simulink model "Rasmusson"  (R2021b)
settings: Solver=ode15s  StartTime=0.0  StopTime=200  FixedStep=1e-4  MaxStep=0.1  RelTol=1e-6  EnableMultiTasking=on
values from neighbouring files (symbols this model uses):
  Acap = 1.534e-4    (= 0.0001534)    [solver.m]
  aKss = 0.417069e-3    (= 0.000417069)    [solver.m]
  ato_f = 0.265563e-2    (= 0.00265563)    [solver.m]
  ato_s = 0.417069e-3    (= 0.000417069)    [solver.m]
  aur = 0.417069e-3    (= 0.000417069)    [solver.m]
  C2 = 0.124216e-3    (= 0.000124216)    [solver.m]
  C3 = 0.578679e-8    (= 5.78679e-09)    [solver.m]
  C4 = 0.119816e-12    (= 1.19816e-13)    [solver.m]
  Cai = 0.115001    [solver.m]
  CaJSR = 1299.50    (= 1299.5)    [solver.m]
  CaNSR = 1299.50    (= 1299.5)    [solver.m]
  Cao = 1800    [solver.m]
  Cass = 0.115001    [solver.m]
  CK1 = 0.992513e-3    (= 0.000992513)    [solver.m]
  CK2 = 0.641229e-3    (= 0.000641229)    [solver.m]
  Cm = 1.0    (= 1)    [solver.m]
  CMDN_tot = 50.0    (= 50)    [solver.m]
  CNa1 = 0.279132e-3    (= 0.000279132)    [solver.m]
  CNa2 = 0.020752    [solver.m]
  CSQN_tot = 15000.0    (= 15000)    [solver.m]
  ECa_L = 63.0    (= 63)    [solver.m]
  ECl = -40.0    (= -40)    [solver.m]
  F = 96.5    [solver.m]
  GCab = 0.000367    [solver.m]
  GCaL = 0.1729    [solver.m]
  GCl_Ca = 10.0    (= 10)    [solver.m]
  GKr = 0.078    [solver.m]
  GKs = 0.00575    [solver.m]
  GKss = 0.050    (= 0.05)    [solver.m]
  GKtof = pktof(6)    [solver.m]
  GKtos = 0.0    (= 0)    [solver.m]
  GKur = pkslow(6)    [solver.m]
  GNa = 13.0    (= 13)    [solver.m]
  GNab = 0.0026    [solver.m]
  HTRPN_tot = 140.0    (= 140)    [solver.m]
  HTRPNCa = 125.290    (= 125.29)    [solver.m]
  I1 = 0.497923e-18    (= 4.97923e-19)    [solver.m]
  I1Na = 0.673345e-6    (= 6.73345e-07)    [solver.m]
  I2 = 0.345847e-13    (= 3.45847e-14)    [solver.m]
  I2Na = 0.155787e-8    (= 1.55787e-09)    [solver.m]
  I3 = 0.185106e-13    (= 1.85106e-14)    [solver.m]
  ICaL_max = 7.0    (= 7)    [solver.m]
  ICNa2 = 0.0113879    [solver.m]
  ICNa3 = 0.342780    (= 0.34278)    [solver.m]
  IFNa = 0.153176e-3    (= 0.000153176)    [solver.m]
  IK = 0.319129e-4    (= 3.19129e-05)    [solver.m]
  iKss = 1.0    (= 1)    [solver.m]
  INaK_max = 0.88    [solver.m]
  Ip_Ca_max = 1.0    (= 1)    [solver.m]
  ito_f = 0.999977    [solver.m]
  ito_s = 0.998543    [solver.m]
  iur = 0.998543    [solver.m]
  ka1 = 0.006075    [solver.m]
  ka2 = 0.07125    [solver.m]
  kb = 0.036778    [solver.m]
  kb1 = 0.00405    [solver.m]
  kb2 = 0.965    [solver.m]
  kc1 = 0.009    [solver.m]
  kc2 = 0.0008    [solver.m]
  kf = 0.023761    [solver.m]
  khtrpn1 = 0.00237    [solver.m]
  khtrpn2 = 3.2e-5    (= 3.2e-05)    [solver.m]
  Ki = 143720    [solver.m]
  kltrpn1 = 0.0327    [solver.m]
  kltrpn2 = 0.0196    [solver.m]
  Km_Ca = 1380    [solver.m]
  Km_Cl = 10.0    (= 10)    [solver.m]
  Km_CMDN = 0.238    [solver.m]
  Km_CSQN = 800.0    (= 800)    [solver.m]
  Km_Ko = 1500    [solver.m]
  Km_Na = 87500    [solver.m]
  Km_Nai = 21000    [solver.m]
  Km_p_Ca = 0.5    [solver.m]
  Km_up = 0.5    [solver.m]
  kNaCa = 292.8    [solver.m]
  Ko = 5400    [solver.m]
  Kpc_half = 20.0    (= 20)    [solver.m]
  Kpc_max = 0.23324    [solver.m]
  Kpcb = 0.0005    [solver.m]
  ksat = 0.1    [solver.m]
  LTRPN_tot = 70.0    (= 70)    [solver.m]
  LTRPNCa = 11.2684    [solver.m]
  Nai = 14237.1    [solver.m]
  Nao = 140000    [solver.m]
  nKs = 0.262753e-3    (= 0.000262753)    [solver.m]
  nu1 = 4.5    [solver.m]
  nu2 = 1.74e-5    (= 1.74e-05)    [solver.m]
  nu3 = 0.45    [solver.m]
  O = 0.930308e-18    (= 9.30308e-19)    [solver.m]
  OK = 0.175298e-3    (= 0.000175298)    [solver.m]
  ONa = 0.713483e-6    (= 7.13483e-07)    [solver.m]
  PC2 = 0.167740e-3    (= 0.00016774)    [solver.m]
  pkslow = kslow_param_wt(best_KslowWt_idx, :)    [solver.m]
  pktof = to_param_ko(best_toKo_idx, :)    [solver.m]
  PO1 = 0.149102e-4    (= 1.49102e-05)    [solver.m]
  PO2 = 0.951726e-10    (= 9.51726e-11)    [solver.m]
  PRyR = 0.0    (= 0)    [solver.m]
  R = 8.314    [solver.m]
  T = 298    [solver.m]
  tautr = 20.0    (= 20)    [solver.m]
  tauxfer = 8.0    (= 8)    [solver.m]
  V = -50:10:50    [result_analysis.m]    (also in solver.m = -82.4202)
  VJSR = 0.12e-6    (= 1.2e-07)    [solver.m]
  Vmyo = 25.84e-6    (= 2.584e-05)    [solver.m]
  VNSR = 2.098e-6    (= 2.098e-06)    [solver.m]
  Vss = 1.485e-9    (= 1.485e-09)    [solver.m]
  yita = 0.35    [solver.m]
(part 2 of 2)

== system Rasmusson/Concentrations/Caconcentration/Ryanodine_receptors/PO2 ==
  note: A20
  Fcn : Fcn  Expr=u*u*u
  Integrator : Integrator  InitialConditionSource=external  InitialCondition=0.951726e-10
  PO2 : Constant  Value=PO2
  Product : Product  Inputs=3  RndMeth=Zero
  Product1 : Product  RndMeth=Zero
  Subtract : Sum  Inputs=+-
  kb+ : Constant  Value=kb1
  kb- : Constant  Value=kb2
  tag scope: PO2=global
  wires:
  Subtract/1 -> Integrator/1
  Integrator/1 -> [PO2], Product1/2
  Product/1 -> Subtract/1
  Product1/1 -> Subtract/2
  Fcn/1 -> Product/2
  kb+/1 -> Product/1
  [Cass] -> Fcn/1
  [PO1] -> Product/3
  kb-/1 -> Product1/1
  PO2/1 -> Integrator/2

== system Rasmusson/Ionic currents/ICaL/O/C1 ==
  note: A24
  Add : Sum  Inputs=+-------
  Constant : Constant
  tag scope: C1=global
  wires:
  Add/1 -> [C1]
  Constant/1 -> Add/1
  [O] -> Add/2
  [C2] -> Add/3
  [C3] -> Add/4
  [C4] -> Add/5
  [I1] -> Add/6
  [I2] -> Add/7
  [I3] -> Add/8

== system Rasmusson/Ionic currents/ICaL/O/C2 ==
  note: A25
  Add : Sum  Inputs=++--
  C2 : Constant  Value=C2
  Gain : Gain  Gain=4
  Gain1 : Gain  Gain=2
  Gain2 : Gain  Gain=3
  Integrator : Integrator  InitialConditionSource=external  InitialCondition=0.124216e-3
  Product{,1..3} (4 alike) : Product  RndMeth=Zero
  tag scope: C2=global
  wires:
  Add/1 -> Integrator/1
  Gain/1 -> Add/1
  Product/1 -> Gain/1
  [alpha] -> Product/1, Product3/1
  [C1] -> Product/2
  [beta] -> Product1/1, Product2/1
  [C3] -> Product1/2
  Product1/1 -> Gain1/1
  Gain1/1 -> Add/2
  Product2/1 -> Add/3
  Integrator/1 -> [C2], Product2/2, Product3/2
  Product3/1 -> Gain2/1
  Gain2/1 -> Add/4
  C2/1 -> Integrator/2

== system Rasmusson/Ionic currents/ICaL/O/C3 ==
  note: A26
  Add : Sum  Inputs=++--
  C3 : Constant  Value=C3
  Gain : Gain  Gain=3
  Gain1 : Gain  Gain=3
  Gain2 : Gain  Gain=2
  Gain3 : Gain  Gain=2
  Integrator : Integrator  InitialConditionSource=external  InitialCondition=0.578679e-8
  Product{,1..3} (4 alike) : Product  RndMeth=Zero
  tag scope: C3=global
  wires:
  Add/1 -> Integrator/1
  Gain/1 -> Add/1
  Product/1 -> Gain/1
  [alpha] -> Product/1, Product3/1
  [C2] -> Product/2
  [beta] -> Product1/1, Product2/1
  [C4] -> Product1/2
  Product1/1 -> Gain1/1
  Gain1/1 -> Add/2
  Product2/1 -> Gain2/1
  Gain2/1 -> Add/3
  Product3/1 -> Gain3/1
  Gain3/1 -> Add/4
  C3/1 -> Integrator/2
  Integrator/1 -> [C3], Product3/2, Product2/2

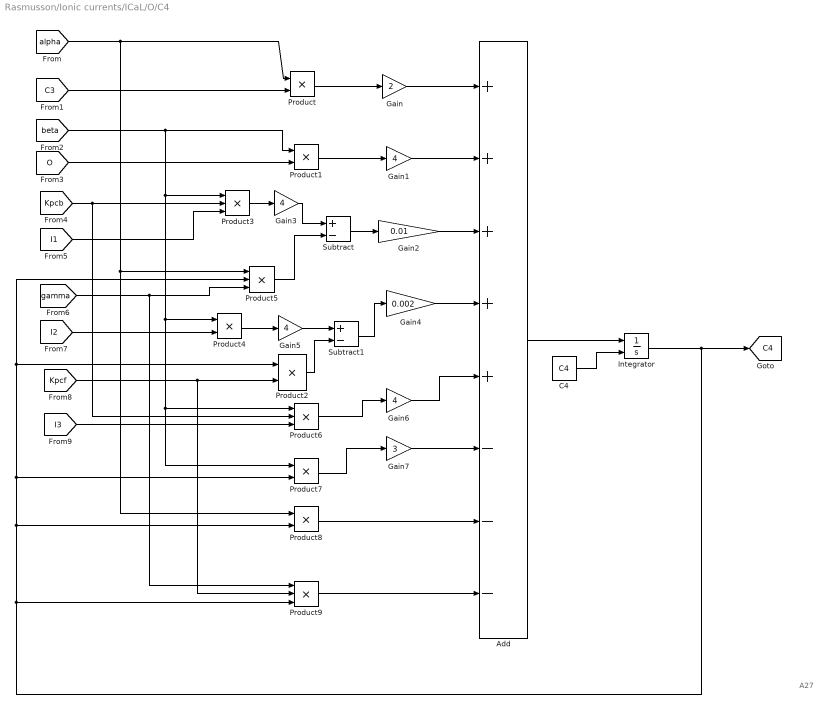
== system Rasmusson/Ionic currents/ICaL/O/C4 ==
  note: A27
  Add : Sum  Inputs=+++++---
  C4 : Constant  Value=C4
  Gain : Gain  Gain=2
  Gain{1,3,5..6} (4 alike) : Gain  Gain=4
  Gain2 : Gain  Gain=0.01
  Gain4 : Gain  Gain=0.002
  Gain7 : Gain  Gain=3
  Integrator : Integrator  InitialConditionSource=external  InitialCondition=0.119816e-12
  Product{,1..2,4,7..8} (6 alike) : Product  RndMeth=Zero
  Product{3,5..6,9} (4 alike) : Product  Inputs=3  RndMeth=Zero
  Subtract : Sum  Inputs=+-
  Subtract1 : Sum  Inputs=+-
  tag scope: C4=global
  wires:
  Integrator/1 -> [C4], Product5/2, Product2/1, Product7/2, Product8/2, Product9/3
  Add/1 -> Integrator/1
  Gain/1 -> Add/1
  Product/1 -> Gain/1
  [alpha] -> Product/1, Product5/1, Product8/1
  [C3] -> Product/2
  Gain1/1 -> Add/2
  Product1/1 -> Gain1/1
  [beta] -> Product1/1, Product3/1, Product4/1, Product6/1, Product7/1
  [O] -> Product1/2
  Subtract/1 -> Gain2/1
  Gain2/1 -> Add/3
  Gain3/1 -> Subtract/1
  Product3/1 -> Gain3/1
  [Kpcb] -> Product3/2, Product6/2
  [I1] -> Product3/3
  Product5/1 -> Subtract/2
  [gamma] -> Product5/3, Product9/1
  Subtract1/1 -> Gain4/1
  Gain5/1 -> Subtract1/1
  Product4/1 -> Gain5/1
  [I2] -> Product4/2
  Product2/1 -> Subtract1/2
  [Kpcf] -> Product2/2, Product9/2
  Gain6/1 -> Add/5
  Product6/1 -> Gain6/1
  Gain4/1 -> Add/4
  [I3] -> Product6/3
  Gain7/1 -> Add/6
  Product7/1 -> Gain7/1
  Product8/1 -> Add/7
  Product9/1 -> Add/8
  C4/1 -> Integrator/2

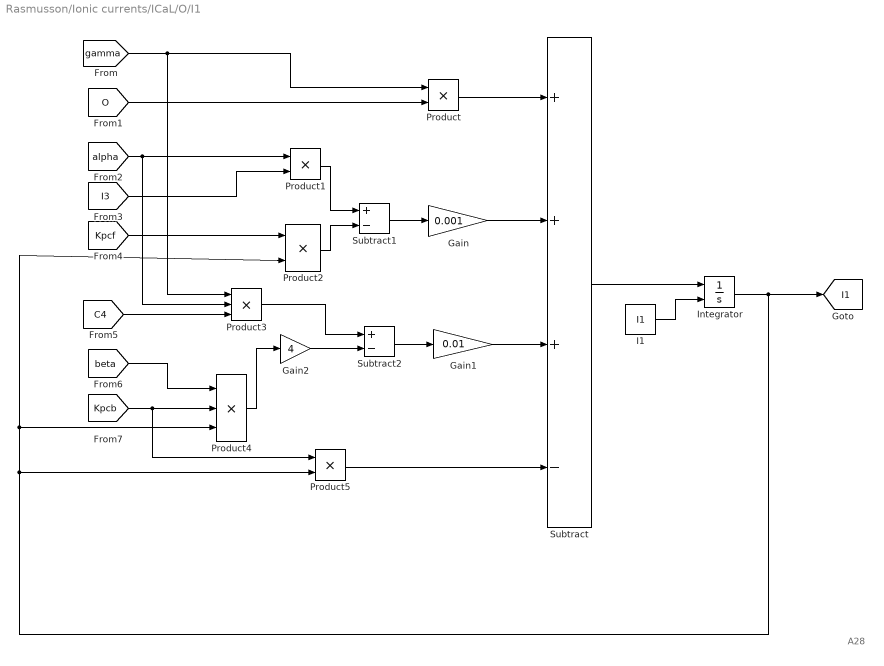
== system Rasmusson/Ionic currents/ICaL/O/I1 ==
  note: A28
  Gain : Gain  Gain=0.001
  Gain1 : Gain  Gain=0.01
  Gain2 : Gain  Gain=4
  I1 : Constant  Value=I1
  Integrator : Integrator  InitialConditionSource=external  InitialCondition=0.497923e-18
  Product{,1..2,5} (4 alike) : Product  RndMeth=Zero
  Product3 : Product  Inputs=3  RndMeth=Zero
  Product4 : Product  Inputs=3  RndMeth=Zero
  Subtract : Sum  Inputs=+++-
  Subtract1 : Sum  Inputs=+-
  Subtract2 : Sum  Inputs=+-
  tag scope: I1=global
  wires:
  Subtract/1 -> Integrator/1
  [gamma] -> Product/1, Product3/1
  [O] -> Product/2
  Product/1 -> Subtract/1
  Gain/1 -> Subtract/2
  Subtract1/1 -> Gain/1
  Integrator/1 -> [I1], Product2/2, Product4/3, Product5/2
  [alpha] -> Product1/1, Product3/2
  Product1/1 -> Subtract1/1
  Product2/1 -> Subtract1/2
  [I3] -> Product1/2
  [Kpcf] -> Product2/1
  Gain1/1 -> Subtract/3
  Subtract2/1 -> Gain1/1
  Gain2/1 -> Subtract2/2
  Product3/1 -> Subtract2/1
  Product4/1 -> Gain2/1
  [C4] -> Product3/3
  [beta] -> Product4/1
  [Kpcb] -> Product4/2, Product5/1
  Product5/1 -> Subtract/4
  I1/1 -> Integrator/2

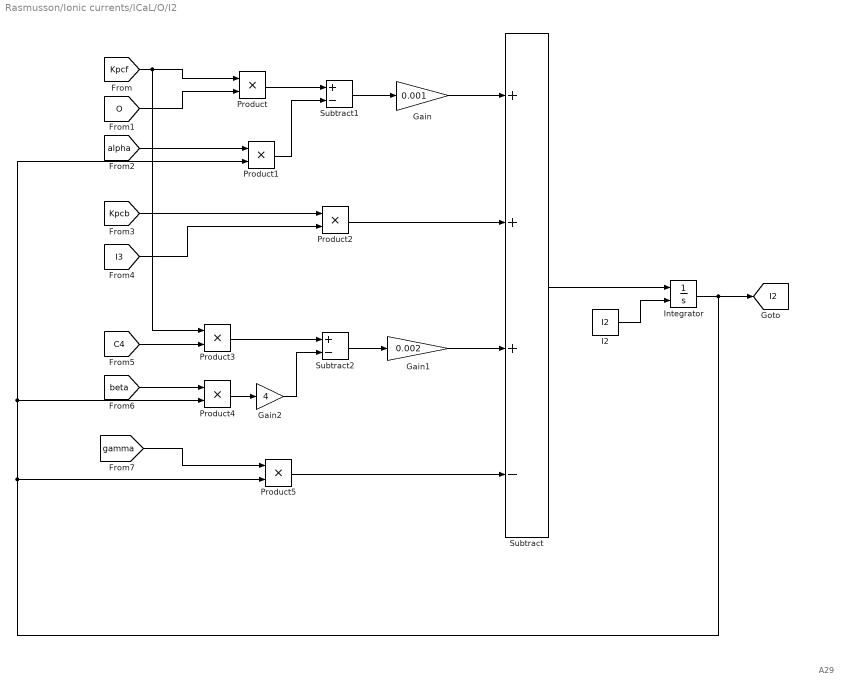
== system Rasmusson/Ionic currents/ICaL/O/I2 ==
  note: A29
  Gain : Gain  Gain=0.001
  Gain1 : Gain  Gain=0.002
  Gain2 : Gain  Gain=4
  I2 : Constant  Value=I2
  Integrator : Integrator  InitialConditionSource=external  InitialCondition=0.345847e-13
  Product{,1..5} (6 alike) : Product  RndMeth=Zero
  Subtract : Sum  Inputs=+++-
  Subtract1 : Sum  Inputs=+-
  Subtract2 : Sum  Inputs=+-
  tag scope: I2=global
  wires:
  Integrator/1 -> [I2], Product1/2, Product4/2, Product5/2
  Product1/1 -> Subtract1/2
  Product/1 -> Subtract1/1
  Subtract1/1 -> Gain/1
  [Kpcf] -> Product/1, Product3/1
  [O] -> Product/2
  [alpha] -> Product1/1
  Product2/1 -> Subtract/2
  [Kpcb] -> Product2/1
  [I3] -> Product2/2
  Product4/1 -> Gain2/1
  Gain2/1 -> Subtract2/2
  Subtract2/1 -> Gain1/1
  Product3/1 -> Subtract2/1
  [C4] -> Product3/2
  [beta] -> Product4/1
  [gamma] -> Product5/1
  Product5/1 -> Subtract/4
  Gain1/1 -> Subtract/3
  Gain/1 -> Subtract/1
  Subtract/1 -> Integrator/1
  I2/1 -> Integrator/2

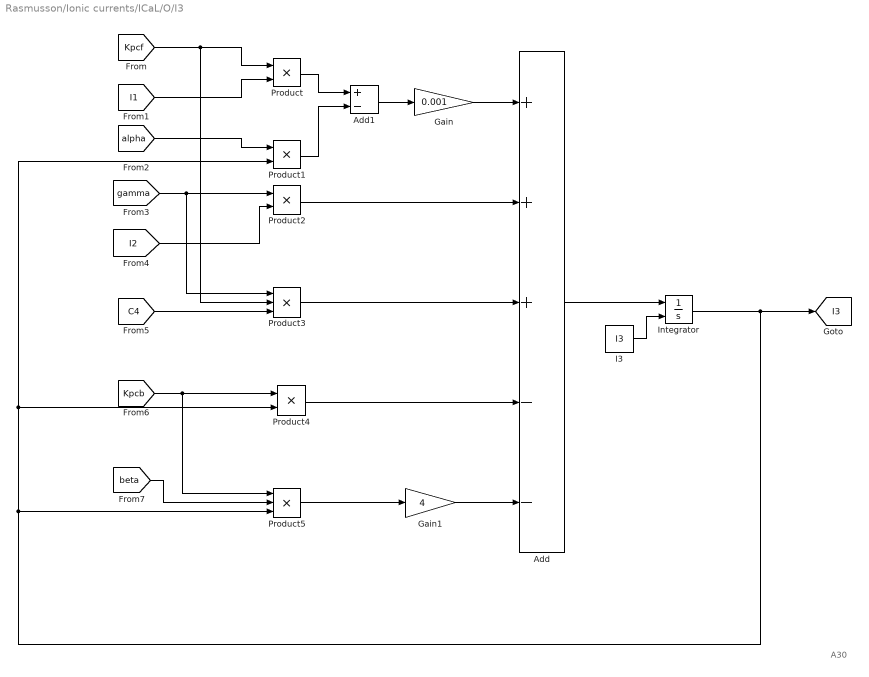
== system Rasmusson/Ionic currents/ICaL/O/I3 ==
  note: A30
  Add : Sum  Inputs=+++--
  Add1 : Sum  Inputs=+-
  Gain : Gain  Gain=0.001
  Gain1 : Gain  Gain=4
  I3 : Constant  Value=I3
  Integrator : Integrator  InitialConditionSource=external  InitialCondition=0.185106e-13
  Product{,1..2,4} (4 alike) : Product  RndMeth=Zero
  Product3 : Product  Inputs=3  RndMeth=Zero
  Product5 : Product  Inputs=3  RndMeth=Zero
  tag scope: I3=global
  wires:
  Integrator/1 -> [I3], Product1/2, Product4/2, Product5/3
  Add/1 -> Integrator/1
  Gain/1 -> Add/1
  Add1/1 -> Gain/1
  [alpha] -> Product1/1
  [I1] -> Product/2
  [Kpcf] -> Product/1, Product3/2
  Product/1 -> Add1/1
  Product1/1 -> Add1/2
  [gamma] -> Product2/1, Product3/1
  [I2] -> Product2/2
  Product2/1 -> Add/2
  Product3/1 -> Add/3
  [C4] -> Product3/3
  Product4/1 -> Add/4
  [Kpcb] -> Product4/1, Product5/1
  Product5/1 -> Gain1/1
  [beta] -> Product5/2
  I3/1 -> Integrator/2
  Gain1/1 -> Add/5

== system Rasmusson/Ionic currents/ICaL/O/Kpcb ==
  Kpcb : Constant  Value=Kpcb
  tag scope: Kpcb=global
  wires:
  Kpcb/1 -> [Kpcb]

== system Rasmusson/Ionic currents/ICaL/O/Kpcf ==
  note: A34
  Kpcf : Fcn  Expr=13*(1-exp(-(u+14.5)*(u+14.5)/100))
  tag scope: Kpcf=global
  wires:
  [volt] -> Kpcf/1
  Kpcf/1 -> [Kpcf]

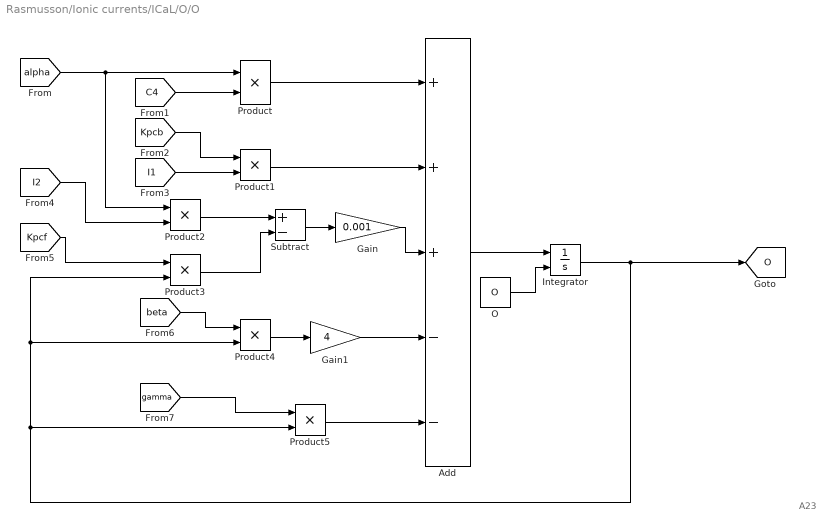
== system Rasmusson/Ionic currents/ICaL/O/O ==
  note: A23
  Add : Sum  Inputs=+++--
  Gain : Gain  Gain=0.001
  Gain1 : Gain  Gain=4
  Integrator : Integrator  InitialConditionSource=external  InitialCondition=0.930308e-18
  O : Constant  Value=O
  Product{,1..5} (6 alike) : Product  RndMeth=Zero
  Subtract : Sum  Inputs=+-
  tag scope: O=global
  wires:
  Add/1 -> Integrator/1
  Integrator/1 -> [O], Product3/2, Product4/2, Product5/2
  Product/1 -> Add/1
  [alpha] -> Product/1, Product2/1
  [C4] -> Product/2
  Product1/1 -> Add/2
  [Kpcb] -> Product1/1
  [I1] -> Product1/2
  Gain/1 -> Add/3
  Subtract/1 -> Gain/1
  Product2/1 -> Subtract/1
  Product3/1 -> Subtract/2
  [I2] -> Product2/2
  [Kpcf] -> Product3/1
  Gain1/1 -> Add/4
  Product4/1 -> Gain1/1
  [beta] -> Product4/1
  Product5/1 -> Add/5
  [gamma] -> Product5/1
  O/1 -> Integrator/2

== system Rasmusson/Ionic currents/ICaL/O/alpha ==
  note: A31
  alpha : Fcn  Expr=(0.4*exp((u+12)/10)*(1+0.7*exp(-(u+40)*(u+40)/10)-0.75*exp(-(u+20)*(u+20)/400)))/(1+0.12*exp((u+12)/10))
  tag scope: alpha=global
  wires:
  alpha/1 -> [alpha]
  [volt] -> alpha/1

== system Rasmusson/Ionic currents/ICaL/O/beta ==
  note: A32
  beta : Fcn  Expr=0.05*exp(-(u+12)/13)
  tag scope: beta=global
  wires:
  [volt] -> beta/1
  beta/1 -> [beta]

== system Rasmusson/Ionic currents/ICaL/O/gamma ==
  note: A33
  Divide : Product  Inputs=**/
  Kpchalf : Constant  Value=Kpc_half
  Kpcmax : Constant  Value=Kpc_max
  Subtract : Sum
  tag scope: gamma=global
  wires:
  Divide/1 -> [gamma]
  Kpcmax/1 -> Divide/1
  [Cass] -> Divide/2, Subtract/1
  Subtract/1 -> Divide/3
  Kpchalf/1 -> Subtract/2

== system Rasmusson/Ionic currents/INa/ONa/CNa1 ==
  note: A44
  Add : Sum  Inputs=+++---
  CNa1 : Constant  Value=CNa1
  Integrator : Integrator  InitialConditionSource=external  InitialCondition=0.279132e-3
  Product{,1..5} (6 alike) : Product  RndMeth=Zero
  tag scope: CNa1=global
  wires:
  [betaNa3] -> Product5/1
  [alphaNa13] -> Product4/1
  [betaNa12] -> Product3/1
  [IFNa] -> Product2/2
  [alphaNa3] -> Product2/1
  [ONa] -> Product1/2
  [betaNa13] -> Product1/1
  [CNa2] -> Product/2
  [alphaNa12] -> Product/1
  Product5/1 -> Add/6
  Product4/1 -> Add/5
  Product3/1 -> Add/4
  Product2/1 -> Add/3
  Product1/1 -> Add/2
  Product/1 -> Add/1
  Add/1 -> Integrator/1
  Integrator/1 -> Product5/2, Product4/2, Product3/2, [CNa1]
  CNa1/1 -> Integrator/2

== system Rasmusson/Ionic currents/INa/ONa/CNa2 ==
  note: A43
  Add : Sum  Inputs=+++---
  CNa2 : Constant  Value=CNa2
  Integrator : Integrator  InitialConditionSource=external  InitialCondition=0.020752
  Product{,1..5} (6 alike) : Product  RndMeth=Zero
  tag scope: CNa2=global
  wires:
  Integrator/1 -> [CNa2], Product3/2, Product4/2, Product5/2
  Add/1 -> Integrator/1
  Product/1 -> Add/1
  Product1/1 -> Add/2
  Product2/1 -> Add/3
  Product3/1 -> Add/4
  Product4/1 -> Add/5
  Product5/1 -> Add/6
  [alphaNa11] -> Product/1
  [CNa3] -> Product/2
  [betaNa12] -> Product1/1
  [CNa1] -> Product1/2
  [alphaNa3] -> Product2/1
  [ICNa2] -> Product2/2
  [betaNa11] -> Product3/1
  [alphaNa12] -> Product4/1
  [betaNa3] -> Product5/1
  CNa2/1 -> Integrator/2

== system Rasmusson/Ionic currents/INa/ONa/CNa3 ==
  note: A42
  Add : Sum  Inputs=+--------
  Constant : Constant
  tag scope: CNa3=global
  wires:
  Add/1 -> [CNa3]
  Constant/1 -> Add/1
  [ONa] -> Add/2
  [CNa1] -> Add/3
  [CNa2] -> Add/4
  [IFNa] -> Add/5
  [I1Na] -> Add/6
  [I2Na] -> Add/7
  [ICNa2] -> Add/8
  [ICNa3] -> Add/9

== system Rasmusson/Ionic currents/INa/ONa/I1Na ==
  note: A47
  Add : Sum  Inputs=++--
  I1Na : Constant  Value=I1Na
  Integrator : Integrator  InitialConditionSource=external  InitialCondition=0.673345e-6
  Product{,1,3,5} (4 alike) : Product  RndMeth=Zero
  tag scope: I1Na=global
  wires:
  Product3/1 -> Add/3
  Product5/1 -> Add/4
  Integrator/1 -> Product5/2, Product3/2, [I1Na]
  Product/1 -> Add/1
  Product1/1 -> Add/2
  [alphaNa5] -> Product5/1
  [betaNa4] -> Product3/1
  [I2Na] -> Product1/2
  [betaNa5] -> Product1/1
  [IFNa] -> Product/2
  [alphaNa4] -> Product/1
  Add/1 -> Integrator/1
  I1Na/1 -> Integrator/2

== system Rasmusson/Ionic currents/INa/ONa/I2Na ==
  note: A48
  Add : Sum  Inputs=+-
  I2Na : Constant  Value=I2Na
  Integrator : Integrator  InitialConditionSource=external  InitialCondition=0.155787e-8
  Product : Product  RndMeth=Zero
  Product5 : Product  RndMeth=Zero
  tag scope: I2Na=global
  wires:
  Add/1 -> Integrator/1
  [alphaNa5] -> Product/1
  [I1Na] -> Product/2
  [betaNa5] -> Product5/1
  Integrator/1 -> [I2Na], Product5/2
  Product5/1 -> Add/2
  Product/1 -> Add/1
  I2Na/1 -> Integrator/2

== system Rasmusson/Ionic currents/INa/ONa/ICNa2 ==
  note: A49
  Add : Sum  Inputs=+++---
  ICNa2 : Constant  Value=ICNa2
  Integrator : Integrator  InitialConditionSource=external  InitialCondition=0.0113879
  Product{,1..5} (6 alike) : Product  RndMeth=Zero
  tag scope: ICNa2=global
  wires:
  [alphaNa3] -> Product5/1
  [alphaNa12] -> Product4/1
  [betaNa11] -> Product3/1
  [CNa2] -> Product2/2
  [betaNa3] -> Product2/1
  [IFNa] -> Product1/2
  [betaNa12] -> Product1/1
  [ICNa3] -> Product/2
  [alphaNa11] -> Product/1
  Product5/1 -> Add/6
  Product4/1 -> Add/5
  Product3/1 -> Add/4
  Product2/1 -> Add/3
  Product1/1 -> Add/2
  Product/1 -> Add/1
  Add/1 -> Integrator/1
  Integrator/1 -> Product5/2, Product4/2, Product3/2, [ICNa2]
  ICNa2/1 -> Integrator/2

== system Rasmusson/Ionic currents/INa/ONa/ICNa3 ==
  note: A50
  Add : Sum  Inputs=++--
  ICNa3 : Constant  Value=ICNa3
  Integrator : Integrator  InitialConditionSource=external  InitialCondition=0.342780
  Product{,1,3,5} (4 alike) : Product  RndMeth=Zero
  tag scope: ICNa3=global
  wires:
  Add/1 -> Integrator/1
  [betaNa11] -> Product/1
  [ICNa2] -> Product/2
  [betaNa3] -> Product1/1
  [CNa3] -> Product1/2
  [alphaNa11] -> Product3/1
  [alphaNa3] -> Product5/1
  Product1/1 -> Add/2
  Product/1 -> Add/1
  Integrator/1 -> [ICNa3], Product3/2, Product5/2
  Product5/1 -> Add/4
  Product3/1 -> Add/3
  ICNa3/1 -> Integrator/2

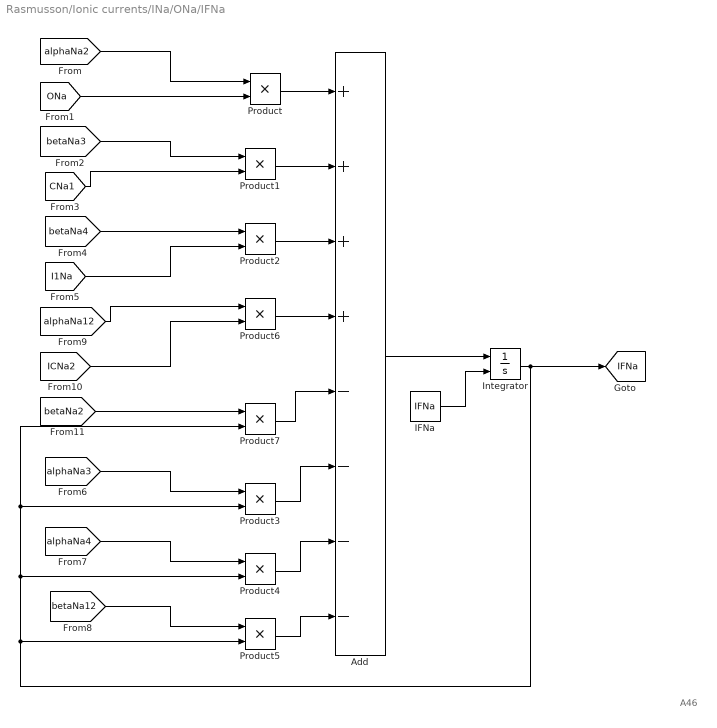
== system Rasmusson/Ionic currents/INa/ONa/IFNa ==
  note: A46
  Add : Sum  Inputs=++++----
  IFNa : Constant  Value=IFNa
  Integrator : Integrator  InitialConditionSource=external  InitialCondition=0.153176e-3
  Product{,1..7} (8 alike) : Product  RndMeth=Zero
  tag scope: IFNa=global
  wires:
  [betaNa12] -> Product5/1
  [alphaNa4] -> Product4/1
  [alphaNa3] -> Product3/1
  [I1Na] -> Product2/2
  [betaNa4] -> Product2/1
  [CNa1] -> Product1/2
  [betaNa3] -> Product1/1
  [ONa] -> Product/2
  [alphaNa2] -> Product/1
  Product2/1 -> Add/3
  Product1/1 -> Add/2
  Product/1 -> Add/1
  Add/1 -> Integrator/1
  Integrator/1 -> Product5/2, Product4/2, Product3/2, Product7/2, [IFNa]
  [ICNa2] -> Product6/2
  [alphaNa12] -> Product6/1
  Product6/1 -> Add/4
  [betaNa2] -> Product7/1
  Product7/1 -> Add/5
  Product3/1 -> Add/6
  Product4/1 -> Add/7
  Product5/1 -> Add/8
  IFNa/1 -> Integrator/2

== system Rasmusson/Ionic currents/INa/ONa/ONa ==
  note: A45
  Add : Sum  Inputs=++--
  Integrator : Integrator  InitialConditionSource=external  InitialCondition=0.713483e-6
  ONa : Constant  Value=ONa
  Product{,1,3,5} (4 alike) : Product  RndMeth=Zero
  tag scope: ONa=global
  wires:
  Add/1 -> Integrator/1
  [alphaNa13] -> Product/1
  [CNa1] -> Product/2
  [betaNa2] -> Product1/1
  [IFNa] -> Product1/2
  [betaNa13] -> Product3/1
  [alphaNa2] -> Product5/1
  Product1/1 -> Add/2
  Product/1 -> Add/1
  Integrator/1 -> [ONa], Product3/2, Product5/2
  Product5/1 -> Add/4
  Product3/1 -> Add/3
  ONa/1 -> Integrator/2

== system Rasmusson/Ionic currents/INa/ONa/alphaNa11 ==
  note: A51
  alphaNa11 : Fcn  Expr=3.802/(0.1027*exp(-(u+2.5)/17)+0.2*exp(-(u+2.5)/150))
  tag scope: alphaNa11=global
  wires:
  [volt] -> alphaNa11/1
  alphaNa11/1 -> [alphaNa11]

== system Rasmusson/Ionic currents/INa/ONa/alphaNa12 ==
  note: A52
  alphaNa12 : Fcn  Expr=3.802/(0.1027*exp(-(u+2.5)/15)+0.23*exp(-(u+2.5)/150))
  tag scope: alphaNa12=global
  wires:
  alphaNa12/1 -> [alphaNa12]
  [volt] -> alphaNa12/1

== system Rasmusson/Ionic currents/INa/ONa/alphaNa13 ==
  note: A53
  alphaNa13 : Fcn  Expr=3.802/(0.1027*exp(-(u+2.5)/12)+0.25*exp(-(u+2.5)/150))
  tag scope: alphaNa13=global
  wires:
  [volt] -> alphaNa13/1
  alphaNa13/1 -> [alphaNa13]

== system Rasmusson/Ionic currents/INa/ONa/alphaNa2 ==
  note: A59
  alphaNa2 : Fcn  Expr=1/(0.188495*exp(-(u+7)/16.6)+0.393956)
  tag scope: alphaNa2=global
  wires:
  alphaNa2/1 -> [alphaNa2]
  [volt] -> alphaNa2/1

== system Rasmusson/Ionic currents/INa/ONa/alphaNa3 ==
  note: A57
  alphaNa3 : Fcn  Expr=7e-7*exp(-(u+7)/7.7)
  tag scope: alphaNa3=global
  wires:
  alphaNa3/1 -> [alphaNa3]
  [volt] -> alphaNa3/1

== system Rasmusson/Ionic currents/INa/ONa/alphaNa4 ==
  note: A61
  Gain : Gain  Gain=0.001
  tag scope: alphaNa4=global
  wires:
  Gain/1 -> [alphaNa4]
  [alphaNa2] -> Gain/1

== system Rasmusson/Ionic currents/INa/ONa/alphaNa5 ==
  note: A63
  Constant : Constant  Value=95000
  Divide : Product  Inputs=*/
  tag scope: alphaNa5=global
  wires:
  Divide/1 -> [alphaNa5]
  [alphaNa2] -> Divide/1
  Constant/1 -> Divide/2

== system Rasmusson/Ionic currents/INa/ONa/betaNa11 ==
  note: A54
  betaNa11 : Fcn  Expr=0.1917*exp(-(u+2.5)/20.3)
  tag scope: betaNa11=global
  wires:
  betaNa11/1 -> [betaNa11]
  [volt] -> betaNa11/1

== system Rasmusson/Ionic currents/INa/ONa/betaNa12 ==
  note: A55
  betaNa12 : Fcn  Expr=0.2*exp(-(u-2.5)/20.3)
  tag scope: betaNa12=global
  wires:
  [volt] -> betaNa12/1
  betaNa12/1 -> [betaNa12]

== system Rasmusson/Ionic currents/INa/ONa/betaNa13 ==
  note: A56
  betaNa13 : Fcn  Expr=0.22*exp(-(u-7.5)/20.3)
  tag scope: betaNa13=global
  wires:
  betaNa13/1 -> [betaNa13]
  [volt] -> betaNa13/1

== system Rasmusson/Ionic currents/INa/ONa/betaNa2 ==
  note: A60
  Divide : Product  Inputs=***//
  tag scope: betaNa2=global
  wires:
  Divide/1 -> [betaNa2]
  [alphaNa13] -> Divide/1
  [alphaNa2] -> Divide/2
  [alphaNa3] -> Divide/3
  [betaNa13] -> Divide/4
  [betaNa3] -> Divide/5

== system Rasmusson/Ionic currents/INa/ONa/betaNa3 ==
  note: A58
  betaNa3 : Fcn  Expr=0.0084+0.00002*(u+7)
  tag scope: betaNa3=global
  wires:
  [volt] -> betaNa3/1
  betaNa3/1 -> [betaNa3]

== system Rasmusson/Ionic currents/INa/ONa/betaNa4 ==
  note: A62
  tag scope: betaNa4=global
  wires:
  [alphaNa3] -> [betaNa4]

== system Rasmusson/Ionic currents/INa/ONa/betaNa5 ==
  note: A64
  Constant : Constant  Value=50
  Divide : Product  Inputs=*/
  tag scope: betaNa5=global
  wires:
  Divide/1 -> [betaNa5]
  [alphaNa3] -> Divide/1
  Constant/1 -> Divide/2

== system Rasmusson/Ionic currents/INaK/fNaK/sigma ==
  note: A110
  Constant : Constant
  Constant1 : Constant  Value=7
  Constant2 : Constant  Value=67300
  Divide : Product  Inputs=*/
  Divide1 : Product  Inputs=*/
  Math Function : Math  SignedPower=on  SaturateOnIntegerOverflow=on
  Nao : Constant  Value=Nao
  Subtract : Sum  Inputs=+-
  tag scope: sigma=global
  wires:
  Divide/1 -> [sigma]
  Constant1/1 -> Divide/2
  Subtract/1 -> Divide/1
  Constant/1 -> Subtract/2
  Math Function/1 -> Subtract/1
  Nao/1 -> Divide1/1
  Constant2/1 -> Divide1/2
  Divide1/1 -> Math Function/1
